simulink model "rocket_1dof_vertical_sim"  (R2026a)
settings: Solver=ode45  StopTime=40
undefined symbols (not defined in the file): magnitude
libraries: simulink x2
settings Model: Creator=metin  LastModifiedBy=metin

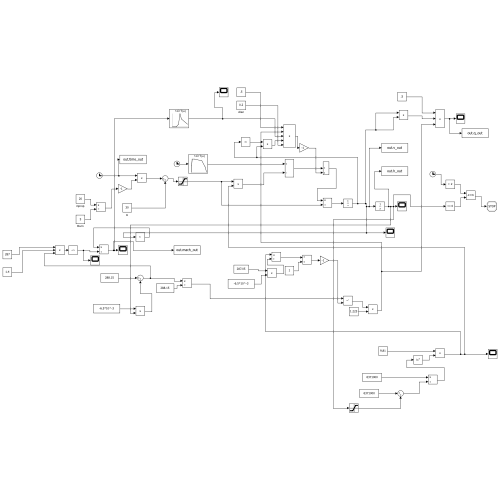
[thumbnail: Simulink's stored preview of the top-level diagram]
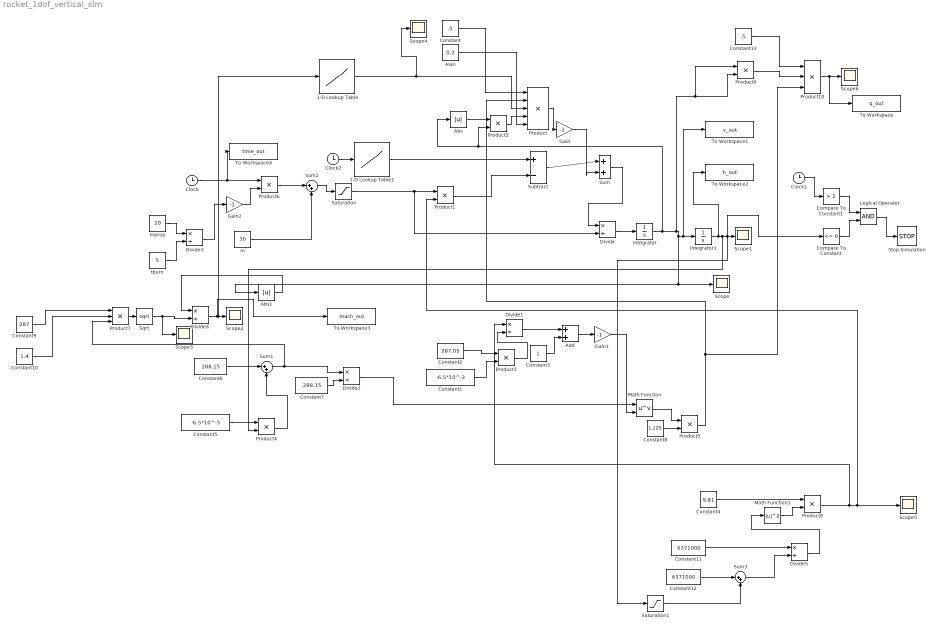
== system rocket_1dof_vertical_sim ==
  1-D Lookup Table : Lookup_n-D  NumberOfTableDimensions=1  BreakpointsForDimension1=[0 0.5 0.8 1.0 1.2 2.0]  Table=[0.4 0.4 0.5 0.9 0.7 0.5]  InternalRulePriority=Speed  RndMeth=Simplest
  1-D Lookup Table1 : Lookup_n-D  NumberOfTableDimensions=1  BreakpointsForDimension1=[0 0.1 0.3 1.0 3.5 4.5 5.0]  Table=[0 800 1500 1500 1300 600 0]  ExtrapMethod=Clip  InternalRulePriority=Speed  RndMeth=Simplest
  Abs : Abs  SaturateOnIntegerOverflow=off
  Abs1 : Abs  SaturateOnIntegerOverflow=off
  Add : Sum
  Alan : Constant  Value=0.2
  Clock : Clock
  Clock1 : Clock
  Clock2 : Clock
  Compare To Constant : simulink/Logic and Bit Operations/Compare To Constant  relop=<=  const=0  OutDataTypeStr=boolean
  Compare To Constant1 : simulink/Logic and Bit Operations/Compare To Constant  relop=>  const=2  OutDataTypeStr=boolean
  Constant : Constant  Value=.5
  Constant1 : Constant  Value=-6.5*10^-3
  Constant10 : Constant  Value=1.4
  Constant11 : Constant  Value=6371000
  Constant12 : Constant  Value=6371000
  Constant13 : Constant  Value=.5
  Constant2 : Constant  Value=287.05
  Constant3 : Constant
  Constant4 : Constant  Value=9.81
  Constant5 : Constant  Value=-6.5*10^-3
  Constant6 : Constant  Value=288.15
  Constant7 : Constant  Value=288.15
  Constant8 : Constant  Value=1.225
  Constant9 : Constant  Value=287
  Divide{,1..5} (6 alike) : Product  Inputs=*/
  Gain : Gain  Gain=-1
  Gain1 : Gain  Gain=-1
  Gain2 : Gain  Gain=-1
  Integrator : Integrator
  Integrator1 : Integrator
  Logical Operator : Logic  AllPortsSameDT=off  OutDataTypeStr=boolean
  Math Function : Math  Operator=pow
  Math Function1 : Math  Operator=magnitude^2
  Product : Product  Inputs=5
  Product{1..6,8..9} (8 alike) : Product
  Product10 : Product  Inputs=3
  Product7 : Product  Inputs=3
  Saturation : Saturate  UpperLimit=50  LowerLimit=20
  Saturation1 : Saturate  UpperLimit=+inf  LowerLimit=0
  Scope{,1..6} (7 alike) : Scope
      Scope settings: ActiveDisplayYMinimum=-1040.0632030836923  ActiveDisplayYMaximum=1500.6195065432053
      Scope1 settings: ActiveDisplayYMinimum=-17244.115733117069  ActiveDisplayYMaximum=4516.1808099883183
      Scope2 settings: ActiveDisplayYMinimum=-0.22441718458003912  ActiveDisplayYMaximum=1.1966346586975363  DataLoggingVariableName=ScopeData2
      Scope3 settings: ActiveDisplayYMinimum=-1  ActiveDisplayYMaximum=1  DataLoggingVariableName=ScopeData3
      Scope4 settings: ActiveDisplayYMinimum=0.36802253137987051  ActiveDisplayYMaximum=0.49017022725327947  DataLoggingVariableName=ScopeData4
      Scope5 settings: ActiveDisplayYMinimum=9.80591248383698  ActiveDisplayYMaximum=9.8092587662830724  DataLoggingVariableName=ScopeData5
      Scope6 settings: ActiveDisplayYMinimum=-11567.923155289805  ActiveDisplayYMaximum=39634.984835919589  DataLoggingVariableName=ScopeData6
  Sqrt : Sqrt
  Stop Simulation : Stop
  Subtract : Sum  Inputs=+-
  Sum{,1..3} (4 alike) : Sum  Inputs=|++
  To Workspace : ToWorkspace  VariableName=q_out  SaveFormat=Timeseries  SampleTime=-1
  To Workspace1 : ToWorkspace  VariableName=v_out  SaveFormat=Timeseries  SampleTime=-1
  To Workspace2 : ToWorkspace  VariableName=h_out  SaveFormat=Timeseries  SampleTime=-1
  To Workspace3 : ToWorkspace  VariableName=mach_out  SaveFormat=Timeseries  SampleTime=-1
  To Workspace4 : ToWorkspace  VariableName=time_out  SaveFormat=Timeseries  SampleTime=-1
  m : Constant  Value=30
  mprop : Constant  Value=20
  tburn : Constant  Value=5
  wires:
  m/1 -> Sum2/2
  Product8/1 -> Divide1/1, Product1/2, Scope5/1
  1-D Lookup Table1/1 -> Subtract/1
  Product1/1 -> Subtract/2
  Saturation/1 -> Divide/2, Product1/1
  Divide/1 -> Integrator/1
  Subtract/1 -> Sum/1
  Sum/1 -> Divide/1
  Constant/1 -> Product/1
  Abs/1 -> Product2/1
  1-D Lookup Table/1 -> Scope4/1, Product/3
  Alan/1 -> Product/5
  Product/1 -> Gain/1
  Product2/1 -> Product/4
  Gain/1 -> Sum/2
  Constant2/1 -> Product3/1
  Constant1/1 -> Product3/2
  Product3/1 -> Divide1/2
  Divide1/1 -> Add/1
  Constant3/1 -> Add/2
  Add/1 -> Gain1/1
  Constant6/1 -> Sum1/1
  Constant5/1 -> Product4/1
  Product4/1 -> Sum1/2
  Sum1/1 -> Product7/3, Divide2/1
  Constant7/1 -> Divide2/2
  Divide2/1 -> Math Function/1
  Gain1/1 -> Math Function/2
  Math Function/1 -> Product5/1
  Constant8/1 -> Product5/2
  Integrator1/1 -> To Workspace2/1, Product4/2, Compare To Constant/1, Saturation1/1, Scope1/1
  Product5/1 -> Product10/3, Product/2
  mprop/1 -> Divide3/1
  tburn/1 -> Divide3/2
  Divide3/1 -> Gain2/1
  Clock/1 -> To Workspace4/1, Product6/1
  Gain2/1 -> Product6/2
  Product6/1 -> Sum2/1
  Sum2/1 -> Saturation/1
  Constant9/1 -> Product7/1
  Constant10/1 -> Product7/2
  Product7/1 -> Sqrt/1
  Sqrt/1 -> Divide4/2, Scope3/1
  Divide4/1 -> To Workspace3/1, 1-D Lookup Table/1, Scope2/1
  Abs1/1 -> Divide4/1
  Constant12/1 -> Sum3/1
  Constant4/1 -> Product8/1
  Sum3/1 -> Divide5/2
  Constant11/1 -> Divide5/1
  Divide5/1 -> Math Function1/1
  Math Function1/1 -> Product8/2
  Saturation1/1 -> Sum3/2
  Integrator/1 -> Product9/1, Product9/2, Abs1/1, Scope/1, To Workspace1/1, Integrator1/1, Abs/1, Product2/2
  Constant13/1 -> Product10/1
  Product9/1 -> Product10/2
  Product10/1 -> To Workspace/1, Scope6/1
  Compare To Constant/1 -> Logical Operator/2
  Clock1/1 -> Compare To Constant1/1
  Compare To Constant1/1 -> Logical Operator/1
  Logical Operator/1 -> Stop Simulation/1
  Clock2/1 -> 1-D Lookup Table1/1
